simulink model "upDownCounter"  (R2022b)
settings: Solver=VariableStepAuto  StartTime=0.0  StopTime=300  RelTol=1e-3
libraries: hdlsllib x2, simulink x1
settings Model: Creator=BAYINDIR  LastModifiedBy=BAYINDIR

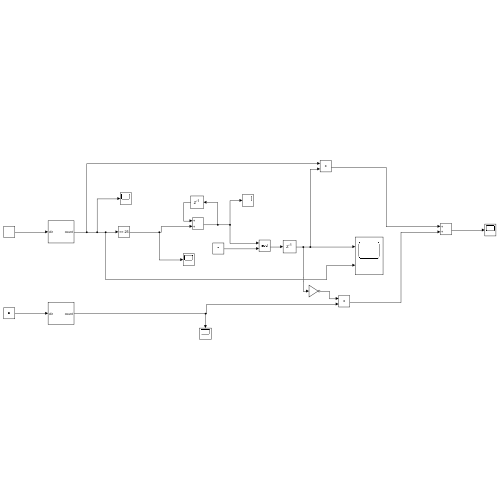
[thumbnail: Simulink's stored preview of the top-level diagram]
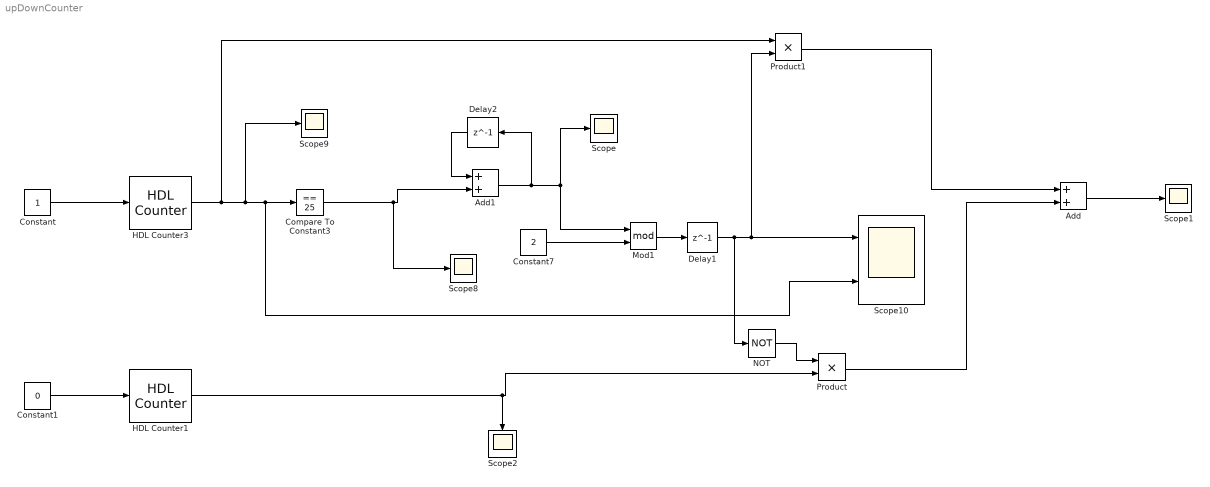
== system upDownCounter ==
  Add : Sum
  Add1 : Sum
  Compare To Constant3 : simulink/Logic and Bit Operations/Compare To Constant  relop===  const=25  OutDataTypeStr=boolean
  Constant : Constant  OutDataTypeStr=boolean  SampleTime=1
  Constant1 : Constant  Value=0  OutDataTypeStr=boolean  SampleTime=1
  Constant7 : Constant  Value=2  OutDataTypeStr=uint32
  Delay1 : Delay  DelayLength=1
  Delay2 : Delay  DelayLength=1
  HDL Counter1 : hdlsllib/Sources/HDL Counter  CountType=Count limited  CountInit=25  CountStep=1  CountMax=0  CountFromType=Initial value  CountFrom=25  CountResetPort=off  CountLoadPort=off  CountEnbPort=off  CountDirPort=on  CountHitOutputPort=off  CountDataType=Unsigned  CountWordLen=32  CountFracLen=0  CountSampTime=1
  HDL Counter3 : hdlsllib/Sources/HDL Counter  CountType=Count limited  CountInit=0  CountStep=1  CountMax=25  CountFromType=Initial value  CountFrom=0  CountResetPort=off  CountLoadPort=off  CountEnbPort=off  CountDirPort=on  CountHitOutputPort=off  CountDataType=Unsigned  CountWordLen=32  CountFracLen=0  CountSampTime=1
  Mod1 : Math  Operator=mod
  NOT : Logic  Operator=NOT  IconShape=distinctive  AllPortsSameDT=off  OutDataTypeStr=boolean
  Product : Product
  Product1 : Product
  Scope{,1..2,8..9} (5 alike) : Scope
  Scope10 : Scope  NumInputPorts=2
  wires:
  HDL Counter3/1 -> Product1/1, Scope9/1, Scope10/2, Compare To Constant3/1
  Delay2/1 -> Add1/1
  Compare To Constant3/1 -> Scope8/1, Add1/2
  Mod1/1 -> Delay1/1
  Constant7/1 -> Mod1/2
  Add1/1 -> Delay2/1, Scope/1, Mod1/1
  Delay1/1 -> NOT/1, Product1/2, Scope10/1
  Constant/1 -> HDL Counter3/1
  Constant1/1 -> HDL Counter1/1
  NOT/1 -> Product/1
  HDL Counter1/1 -> Product/2, Scope2/1
  Product1/1 -> Add/1
  Product/1 -> Add/2
  Add/1 -> Scope1/1
